simulink model "Proiect_PID_Discret"  (R2018b)
settings: Solver=VariableStepAuto  StartTime=0.0  StopTime=30.00  RelTol=1e-3
settings Model: Creator=Nathan  LastModifiedBy=Nathan

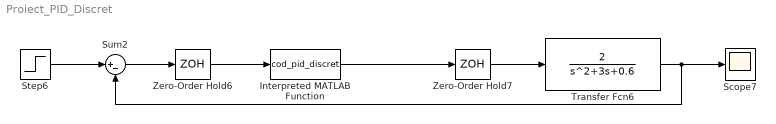
== system Proiect_PID_Discret ==
  Interpreted MATLAB Function : MATLABFcn  MATLABFcn=cod_pid_discret  OutputDimensions=1
  Scope7 : Scope
  Step6 : Step  Time=0  After=7  SampleTime=0
  Sum2 : Sum  Inputs=|+-
  Transfer Fcn6 : TransferFcn  Numerator=2  Denominator=[1 3 0.6]
  Zero-Order Hold6 : ZeroOrderHold  SampleTime=0.005
  Zero-Order Hold7 : ZeroOrderHold  SampleTime=0.005
  wires:
  Step6/1 -> Sum2/1
  Sum2/1 -> Zero-Order Hold6/1
  Zero-Order Hold6/1 -> Interpreted MATLAB Function/1
  Zero-Order Hold7/1 -> Transfer Fcn6/1
  Transfer Fcn6/1 -> Sum2/2, Scope7/1
  Interpreted MATLAB Function/1 -> Zero-Order Hold7/1
